simulink model "HW2d5b"  (R2023b)
settings: Solver=VariableStepAuto  StartTime=0.0  StopTime=10.0  RelTol=1e-3
settings Model: Creator=wureb  LastModifiedBy=Rebing Wu

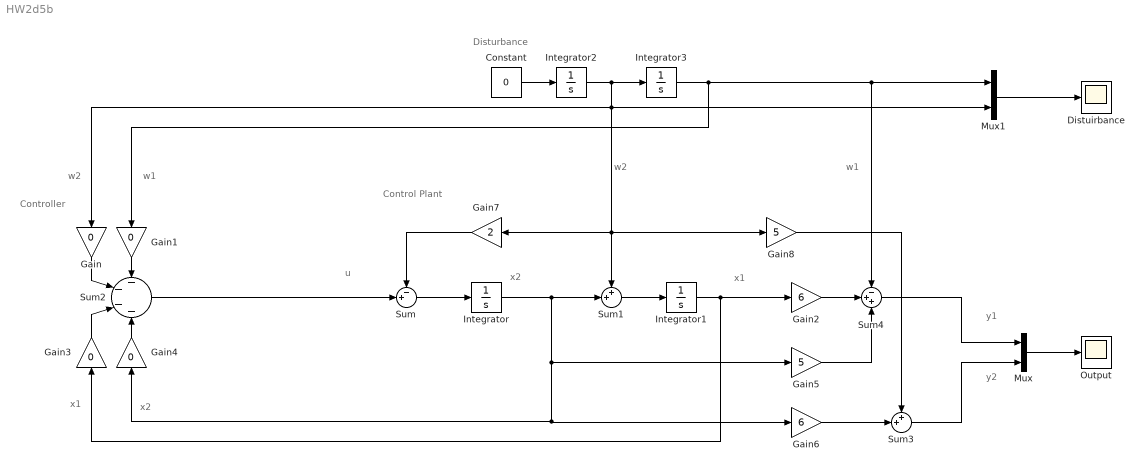
== system HW2d5b ==
  note: Control Plant
  note: Controller
  note: Disturbance
  note: y1
  note: x1
  note: x1
  note: w2
  note: x2
  note: y2
  note: u
  note: w2
  note: w1
  note: x2
  note: w1
  Constant : Constant  Value=0
  Distuirbance : Scope
  Gain{,1,3..4} (4 alike) : Gain  Gain=0
  Gain2 : Gain  Gain=6
  Gain5 : Gain  Gain=5
  Gain6 : Gain  Gain=6
  Gain7 : Gain  Gain=2
  Gain8 : Gain  Gain=5
  Integrator : Integrator  InitialCondition=1
  Integrator1 : Integrator  InitialCondition=1
  Integrator2 : Integrator
  Integrator3 : Integrator
  Mux : Mux  Inputs=2
  Mux1 : Mux  Inputs=2
  Output : Scope
  Sum : Sum  Inputs=-+|
  Sum1 : Sum  Inputs=++|
  Sum2 : Sum  Inputs=-|-|-|-
  Sum3 : Sum  Inputs=++|
  Sum4 : Sum  Inputs=-++
  wires:
  Constant/1 -> Integrator2/1
  Gain3/1 -> Sum2/3
  Gain4/1 -> Sum2/4
  Gain/1 -> Sum2/2
  Gain1/1 -> Sum2/1
  Mux1/1 -> Distuirbance/1
  Sum4/1 -> Mux/1
  Sum3/1 -> Mux/2
  Integrator1/1 -> Gain3/1, Gain2/1
  Integrator/1 -> Gain4/1, Gain6/1, Gain5/1, Sum1/2
  Integrator3/1 -> Gain1/1, Sum4/1, Mux1/1
  Sum1/1 -> Integrator1/1
  Gain8/1 -> Sum3/1
  Gain5/1 -> Sum4/3
  Integrator2/1 -> Mux1/2, Gain7/1, Gain8/1, Sum1/1, Gain/1, Integrator3/1
  Sum/1 -> Integrator/1
  Gain2/1 -> Sum4/2
  Gain6/1 -> Sum3/2
  Gain7/1 -> Sum/1
  Sum2/1 -> Sum/2
  Mux/1 -> Output/1
